simulink model "undirect_graph_compare_TBG"  (R2020a)
settings: Solver=FixedStepAuto  StartTime=0.0  StopTime=10.0  FixedStep=0.0001  RelTol=1e-3
settings Model: Creator=WangQipeng  LastModifiedBy=WangQipeng

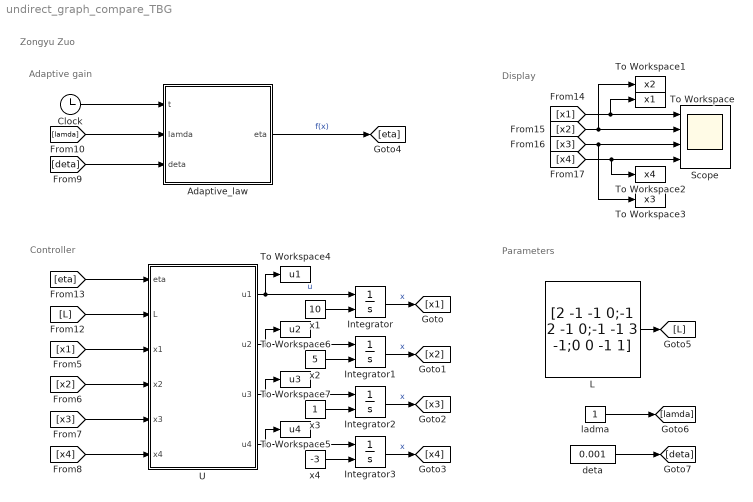
== system undirect_graph_compare_TBG ==
  note: Zongyu Zuo
  note: Controller
  note: Adaptive gain
  note: Display
  note: Parameters
  Adaptive_law : MATLAB Function  TreatAsAtomicUnit=on
  Clock : Clock
  Integrator{,1..3} (4 alike) : Integrator  InitialConditionSource=external  InitialCondition=1
  L : Constant  Value=[2 -1 -1 0;-1 2 -1 0;-1 -1 3 -1;0 0 -1 1]
  Scope : Scope  NumInputPorts=4
  To Workspace : ToWorkspace  VariableName=x1  SaveFormat=Timeseries  SampleTime=-1
  To Workspace1 : ToWorkspace  VariableName=x2  SaveFormat=Timeseries  SampleTime=-1
  To Workspace2 : ToWorkspace  VariableName=x4  SaveFormat=Timeseries  SampleTime=-1
  To Workspace3 : ToWorkspace  VariableName=x3  SaveFormat=Timeseries  SampleTime=-1
  To Workspace4 : ToWorkspace  VariableName=u1  SaveFormat=Timeseries  SampleTime=-1
  To Workspace5 : ToWorkspace  VariableName=u4  SaveFormat=Timeseries  SampleTime=-1
  To Workspace6 : ToWorkspace  VariableName=u2  SaveFormat=Timeseries  SampleTime=-1
  To Workspace7 : ToWorkspace  VariableName=u3  SaveFormat=Timeseries  SampleTime=-1
  U : MATLAB Function  TreatAsAtomicUnit=on
  deta : Constant  Value=0.001
  ladma : Constant
  x1 : Constant  Value=10
  x2 : Constant  Value=5
  x3 : Constant
  x4 : Constant  Value=-3
  wires:
  U/1(u1) -> To Workspace4/1, Integrator/1  "u"
  U/2(u2) -> To Workspace6/1, Integrator1/1
  U/3(u3) -> To Workspace7/1, Integrator2/1
  U/4(u4) -> Integrator3/1, To Workspace5/1
  Integrator/1 -> [x1]  "x"
  Integrator1/1 -> [x2]  "x"
  Integrator2/1 -> [x3]  "x"
  Integrator3/1 -> [x4]  "x"
  [x3] -> U/5(x3)
  [x4] -> U/6(x4)
  [x1] -> U/3(x1)
  [x2] -> U/4(x2)
  L/1 -> [L]
  [deta] -> Adaptive_law/3(deta)
  ladma/1 -> [lamda]
  deta/1 -> [deta]
  [lamda] -> Adaptive_law/2(lamda)
  Clock/1 -> Adaptive_law/1(t)
  [L] -> U/2(L)
  [eta] -> U/1(eta)
  x1/1 -> Integrator/2
  x2/1 -> Integrator1/2
  x3/1 -> Integrator2/2
  x4/1 -> Integrator3/2
  [x1] -> To Workspace/1, Scope/1
  [x2] -> Scope/2, To Workspace1/1
  [x3] -> Scope/3, To Workspace3/1
  [x4] -> Scope/4, To Workspace2/1
  Adaptive_law/1(eta) -> [eta]  "f(x)"

== matlab function undirect_graph_compare_TBG/U ==
  data: eta input; u1 output; L input; x1 input; x2 input; x3 input; x4 input; u2 output; u3 output; u4 output
function [u1,u2,u3,u4] = protocol(eta,L,x1,x2,x3,x4)
x = [x1;x2;x3;x4];
temp = -(eta + 1) * L * x;
u1 = temp(1);
u2 = temp(2);
u3 = temp(3);
u4 = temp(4);

== matlab function undirect_graph_compare_TBG/Adaptive_law ==
  data: t input; eta output; lamda input; deta input
function eta = TBG(t,lamda,deta)
if(t<=4)
    zeta = 10/(4^6)*t^6 - 24/(4^5)*t^5 + 15/(4^4)*t^4;
    d_zeta = 60/(4^6)*t^5 - 120/(4^5)*t^4 + 15/(4^3)*t^3;
else
    zeta = 1;
    d_zeta = 0;
end

eta = d_zeta/(2 * lamda * (1 - zeta + deta));
